simulink model "min_max"  (Simulink 7.4)
settings: Solver=ode45  StartTime=0.0  StopTime=10.0  RelTol=1e-3
libraries: xbsIndex_r4 x38
settings Model: Creator=andryc  LastModifiedBy=andryc

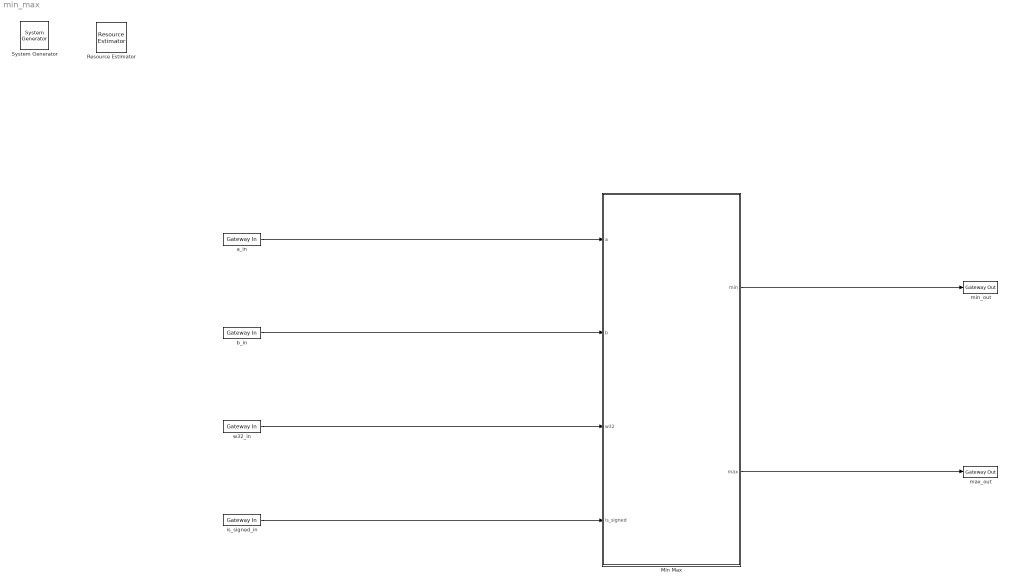
== system min_max ==
  " System Generator" : xbsIndex_r4/ System Generator  Tag=genX  SystemSampleTime=-1  xilinxfamily=virtex5  part=xc5vlx330t  speed=-1  package=ff1738  synthesis_tool=XST  clock_wrapper=Clock Enables  directory=./ngc_netlist  testbench=off  simulink_period=1  sysclk_period=3.333333333  dcm_input_clock_period=10  incr_netlist=off  trim_vbits=Everywhere in SubSystem  dbl_ovrd=According to Block Masks  core_generation=According to Block Masks  run_coregen=off  deprecated_control=off  eval_field=0  block_type=sysgen
  Min Max : Subsystem
  Resource Estimator : xbsIndex_r4/Resource Estimator  Tag=resEstTag  Slices=0  FFs=0  BRAMs=0  LUTs=0  IOBs=0  EBMs=0  TBUFs=0  xl_use_estimator_area=off  est_options=Estimate  block_type=resource_estimator
      settings: AttributesFormatString=Resource\nEstimator
  a_in : xbsIndex_r4/Gateway In  arith_type=Unsigned  n_bits=32  bin_pt=0  quantization=Truncate  overflow=Saturate  period=1  dbl_ovrd=off  timing_constraint=None  locs_specified=off  LOCs={}  hdl_port=on  block_type=gatewayin
      settings: infoedit="Gateway in block.  Converts inputs of type Simulink integer, double and fixed point to  Xilinx fixed point type.<br><br>Hardware notes:  In hardware these blocks become top level input ports."
  b_in : xbsIndex_r4/Gateway In  arith_type=Unsigned  n_bits=32  bin_pt=0  quantization=Truncate  overflow=Saturate  period=1  dbl_ovrd=off  timing_constraint=None  locs_specified=off  LOCs={}  hdl_port=on  block_type=gatewayin
      settings: infoedit="Gateway in block.  Converts inputs of type Simulink integer, double and fixed point to  Xilinx fixed point type.<br><br>Hardware notes:  In hardware these blocks become top level input ports."
  is_signed_in : xbsIndex_r4/Gateway In  arith_type=Unsigned  n_bits=1  bin_pt=0  quantization=Truncate  overflow=Saturate  period=1  dbl_ovrd=off  timing_constraint=None  locs_specified=off  LOCs={}  hdl_port=on  block_type=gatewayin
      settings: infoedit="Gateway in block.  Converts inputs of type Simulink integer, double and fixed point to  Xilinx fixed point type.<br><br>Hardware notes:  In hardware these blocks become top level input ports."
  max_out : xbsIndex_r4/Gateway Out  hdl_port=on  timing_constraint=None  locs_specified=off  LOCs={}  block_type=gatewayout
      settings: infoedit="Gateway out block.  Converts Xilinx fixed point inputs into ouputs of type Simulink integer, double, or fixed point.<br><br>Hardware notes:  In hardware these blocks become top level output ports or are discarded, depending on how they are configured."
  min_out : xbsIndex_r4/Gateway Out  hdl_port=on  timing_constraint=None  locs_specified=off  LOCs={}  block_type=gatewayout
      settings: infoedit="Gateway out block.  Converts Xilinx fixed point inputs into ouputs of type Simulink integer, double, or fixed point.<br><br>Hardware notes:  In hardware these blocks become top level output ports or are discarded, depending on how they are configured."
  w32_in : xbsIndex_r4/Gateway In  arith_type=Unsigned  n_bits=1  bin_pt=0  quantization=Truncate  overflow=Saturate  period=1  dbl_ovrd=off  timing_constraint=None  locs_specified=off  LOCs={}  hdl_port=on  block_type=gatewayin
      settings: infoedit="Gateway in block.  Converts inputs of type Simulink integer, double and fixed point to  Xilinx fixed point type.<br><br>Hardware notes:  In hardware these blocks become top level input ports."
  wires:
  a_in/1 -> Min Max/1(a)
  b_in/1 -> Min Max/2(b)
  w32_in/1 -> Min Max/3(w32)
  is_signed_in/1 -> Min Max/4(is_signed)
  Min Max/2(max) -> max_out/1
  Min Max/1(min) -> min_out/1

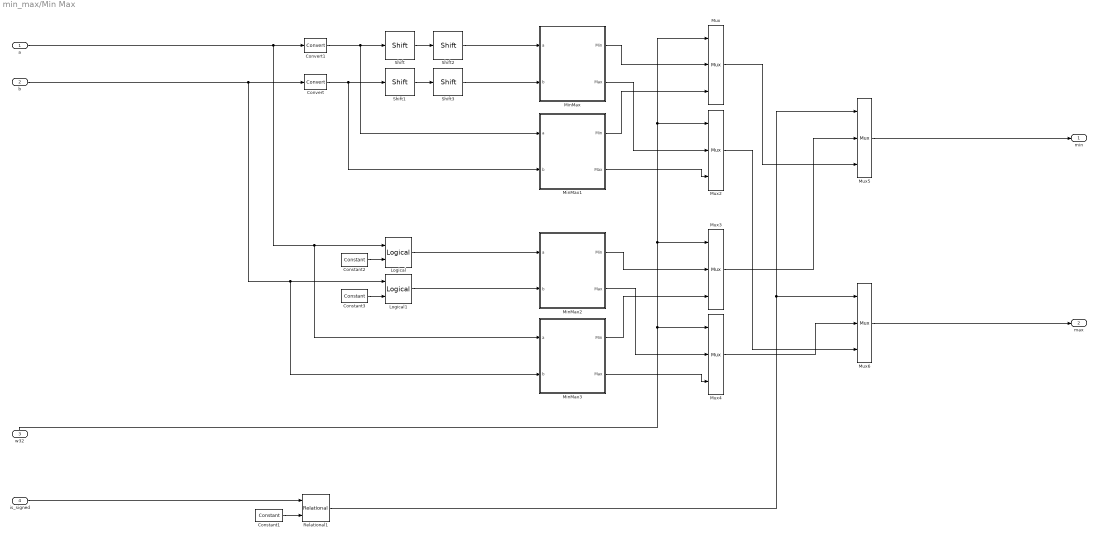
== system min_max/Min Max ==
  a : Inport
  b : Inport  Port=2
  w32 : Inport  Port=3
  is_signed : Inport  Port=4
  Constant1 : xbsIndex_r4/Constant  arith_type=Unsigned  const=1  n_bits=1  bin_pt=0  explicit_period=off  period=1  equ=P=C  opselect=C  inp2=PCIN>>17  opr=+  inp1=P  carry=CIN  dbl_ovrd=off  block_type=constant
      settings: block_version=12.2
  Constant2 : xbsIndex_r4/Constant  arith_type=Unsigned  const=65535  n_bits=32  bin_pt=0  explicit_period=off  period=1  equ=P=C  opselect=C  inp2=PCIN>>17  opr=+  inp1=P  carry=CIN  dbl_ovrd=off  block_type=constant
      settings: block_version=12.2
  Constant3 : xbsIndex_r4/Constant  arith_type=Unsigned  const=65535  n_bits=32  bin_pt=0  explicit_period=off  period=1  equ=P=C  opselect=C  inp2=PCIN>>17  opr=+  inp1=P  carry=CIN  dbl_ovrd=off  block_type=constant
      settings: block_version=12.2
  Convert : xbsIndex_r4/Convert  arith_type="Signed  (2's comp)"  n_bits=31  bin_pt=0  quantization=Truncate  overflow=Saturate  en=off  latency=0  dbl_ovrd=off  pipeline=off  block_type=convert
      settings: block_version=12.2
  Convert1 : xbsIndex_r4/Convert  arith_type="Signed  (2's comp)"  n_bits=32  bin_pt=0  quantization=Truncate  overflow=Saturate  en=off  latency=0  dbl_ovrd=off  pipeline=off  block_type=convert
      settings: block_version=12.2
  Logical : xbsIndex_r4/Logical  logical_function=AND  inputs=2  en=off  latency=0  precision=User Defined  arith_type=Unsigned  n_bits=32  bin_pt=0  align_bp=on  dbl_ovrd=off  block_type=logical
      settings: block_version=12.2
  Logical1 : xbsIndex_r4/Logical  logical_function=AND  inputs=2  en=off  latency=0  precision=User Defined  arith_type=Unsigned  n_bits=32  bin_pt=0  align_bp=on  dbl_ovrd=off  block_type=logical
      settings: block_version=12.2
  MinMax : Subsystem
  MinMax1 : Subsystem
  MinMax2 : Subsystem
  MinMax3 : Subsystem
  Mux{,2..4} (4 alike) : xbsIndex_r4/Mux  inputs=2  en=off  latency=0  precision=Full  arith_type=Unsigned  n_bits=16  bin_pt=14  quantization=Truncate  overflow=Wrap  dbl_ovrd=off  block_type=mux
      settings: block_version=12.2
  Mux5 : xbsIndex_r4/Mux  inputs=2  en=off  latency=0  precision=User Defined  arith_type="Signed  (2's comp)"  n_bits=32  bin_pt=0  quantization=Truncate  overflow=Saturate  dbl_ovrd=off  block_type=mux
      settings: block_version=12.2
  Mux6 : xbsIndex_r4/Mux  inputs=2  en=off  latency=0  precision=User Defined  arith_type=Unsigned  n_bits=32  bin_pt=0  quantization=Truncate  overflow=Saturate  dbl_ovrd=off  block_type=mux
      settings: block_version=12.2
  Relational1 : xbsIndex_r4/Relational  mode=a=b  en=off  latency=0  dbl_ovrd=off  block_type=relational
      settings: block_version=12.2
  Shift : xbsIndex_r4/Shift  shift_dir=Left  shift_bits=16  en=off  latency=0  precision=Full  arith_type="Signed  (2's comp)"  n_bits=31  bin_pt=0  quantization=Truncate  overflow=Saturate  dbl_ovrd=off  block_type=shift
      settings: block_version=12.2
  Shift1 : xbsIndex_r4/Shift  shift_dir=Left  shift_bits=16  en=off  latency=0  precision=Full  arith_type="Signed  (2's comp)"  n_bits=31  bin_pt=0  quantization=Truncate  overflow=Saturate  dbl_ovrd=off  block_type=shift
      settings: block_version=12.2
  Shift2 : xbsIndex_r4/Shift  shift_dir=Right  shift_bits=16  en=off  latency=0  precision=Full  arith_type="Signed  (2's comp)"  n_bits=31  bin_pt=0  quantization=Truncate  overflow=Saturate  dbl_ovrd=off  block_type=shift
      settings: block_version=12.2
  Shift3 : xbsIndex_r4/Shift  shift_dir=Right  shift_bits=16  en=off  latency=0  precision=Full  arith_type="Signed  (2's comp)"  n_bits=31  bin_pt=0  quantization=Truncate  overflow=Saturate  dbl_ovrd=off  block_type=shift
      settings: block_version=12.2
  min : Outport
  max : Outport  Port=2
  wires:
  Constant1/1 -> Relational1/2
  b/1 -> Convert/1, Logical1/1, MinMax3/2(b)
  a/1 -> Convert1/1, Logical/1, MinMax3/1(a)
  Convert1/1 -> Shift/1, MinMax1/1(a)
  Convert/1 -> Shift1/1, MinMax1/2(b)
  Shift1/1 -> Shift3/1
  Shift/1 -> Shift2/1
  Shift2/1 -> MinMax/1(a)
  Shift3/1 -> MinMax/2(b)
  w32/1 -> Mux/1, Mux2/1, Mux3/1, Mux4/1
  MinMax/1(Min) -> Mux/2
  MinMax1/1(Min) -> Mux/3
  MinMax/2(Max) -> Mux2/2
  MinMax1/2(Max) -> Mux2/3
  Constant2/1 -> Logical/2
  Constant3/1 -> Logical1/2
  Logical/1 -> MinMax2/1(a)
  Logical1/1 -> MinMax2/2(b)
  MinMax2/1(Min) -> Mux3/2
  MinMax3/1(Min) -> Mux3/3
  MinMax2/2(Max) -> Mux4/2
  MinMax3/2(Max) -> Mux4/3
  Relational1/1 -> Mux5/1, Mux6/1
  Mux/1 -> Mux5/3
  Mux2/1 -> Mux6/3
  Mux3/1 -> Mux5/2
  Mux4/1 -> Mux6/2
  Mux5/1 -> min/1
  Mux6/1 -> max/1
  is_signed/1 -> Relational1/1

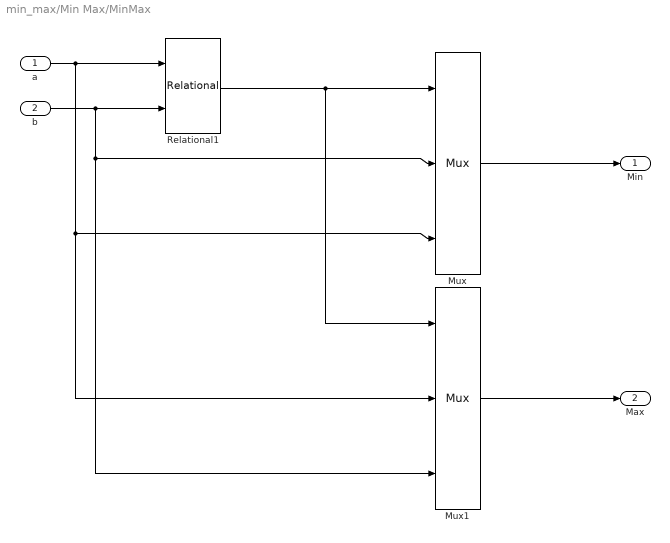
== system min_max/Min Max/MinMax ==
  a : Inport
  b : Inport  Port=2
  Mux : xbsIndex_r4/Mux  inputs=2  en=off  latency=0  precision=Full  arith_type=Unsigned  n_bits=16  bin_pt=14  quantization=Truncate  overflow=Wrap  dbl_ovrd=off  block_type=mux
      settings: block_version=12.2
  Mux1 : xbsIndex_r4/Mux  inputs=2  en=off  latency=0  precision=Full  arith_type=Unsigned  n_bits=16  bin_pt=14  quantization=Truncate  overflow=Wrap  dbl_ovrd=off  block_type=mux
      settings: block_version=12.2
  Relational1 : xbsIndex_r4/Relational  mode=a<=b  en=off  latency=0  dbl_ovrd=off  block_type=relational
      settings: block_version=12.2
  Min : Outport
  Max : Outport  Port=2
  wires:
  Relational1/1 -> Mux/1, Mux1/1
  a/1 -> Relational1/1, Mux/3, Mux1/2
  b/1 -> Relational1/2, Mux/2, Mux1/3
  Mux/1 -> Min/1
  Mux1/1 -> Max/1

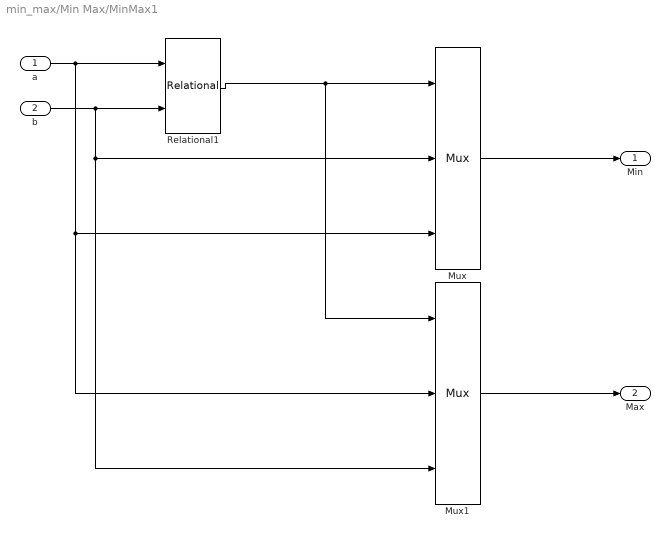
== system min_max/Min Max/MinMax1 ==
  a : Inport
  b : Inport  Port=2
  Mux : xbsIndex_r4/Mux  inputs=2  en=off  latency=0  precision=Full  arith_type=Unsigned  n_bits=16  bin_pt=14  quantization=Truncate  overflow=Wrap  dbl_ovrd=off  block_type=mux
      settings: block_version=12.2
  Mux1 : xbsIndex_r4/Mux  inputs=2  en=off  latency=0  precision=Full  arith_type=Unsigned  n_bits=16  bin_pt=14  quantization=Truncate  overflow=Wrap  dbl_ovrd=off  block_type=mux
      settings: block_version=12.2
  Relational1 : xbsIndex_r4/Relational  mode=a<=b  en=off  latency=0  dbl_ovrd=off  block_type=relational
      settings: block_version=12.2
  Min : Outport
  Max : Outport  Port=2
  wires:
  Mux1/1 -> Max/1
  Mux/1 -> Min/1
  b/1 -> Mux1/3, Mux/2, Relational1/2
  a/1 -> Mux1/2, Mux/3, Relational1/1
  Relational1/1 -> Mux1/1, Mux/1

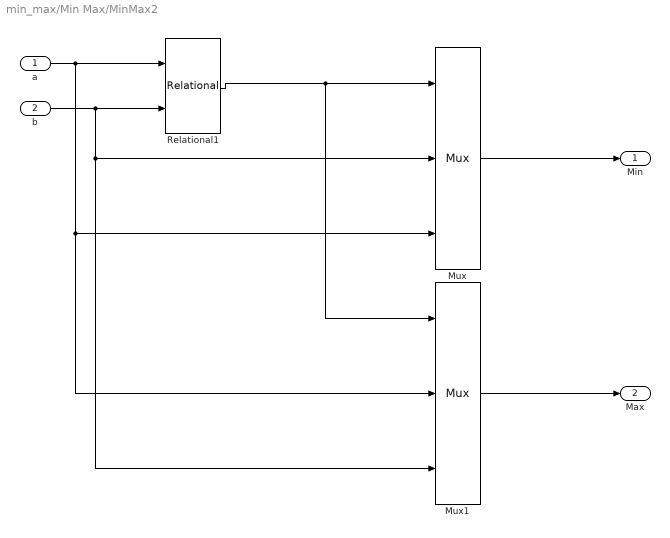
== system min_max/Min Max/MinMax2 ==
  a : Inport
  b : Inport  Port=2
  Mux : xbsIndex_r4/Mux  inputs=2  en=off  latency=0  precision=Full  arith_type=Unsigned  n_bits=16  bin_pt=14  quantization=Truncate  overflow=Wrap  dbl_ovrd=off  block_type=mux
      settings: block_version=12.2
  Mux1 : xbsIndex_r4/Mux  inputs=2  en=off  latency=0  precision=Full  arith_type=Unsigned  n_bits=16  bin_pt=14  quantization=Truncate  overflow=Wrap  dbl_ovrd=off  block_type=mux
      settings: block_version=12.2
  Relational1 : xbsIndex_r4/Relational  mode=a<=b  en=off  latency=0  dbl_ovrd=off  block_type=relational
      settings: block_version=12.2
  Min : Outport
  Max : Outport  Port=2
  wires:
  Relational1/1 -> Mux/1, Mux1/1
  a/1 -> Relational1/1, Mux/3, Mux1/2
  b/1 -> Relational1/2, Mux/2, Mux1/3
  Mux/1 -> Min/1
  Mux1/1 -> Max/1

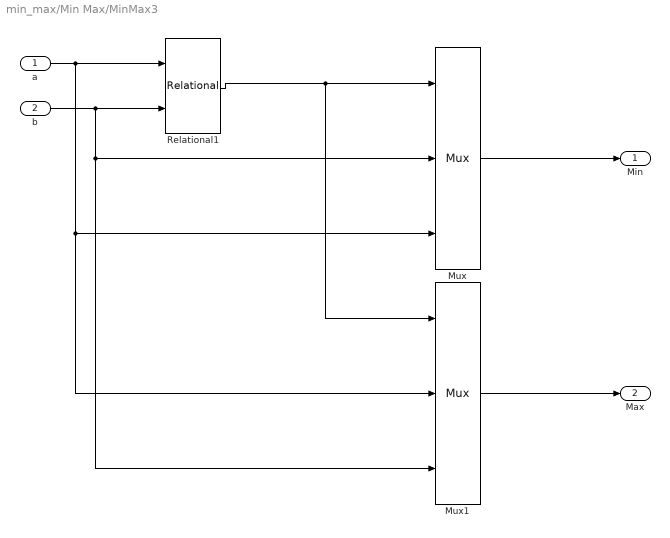
== system min_max/Min Max/MinMax3 ==
  a : Inport
  b : Inport  Port=2
  Mux : xbsIndex_r4/Mux  inputs=2  en=off  latency=0  precision=Full  arith_type=Unsigned  n_bits=16  bin_pt=14  quantization=Truncate  overflow=Wrap  dbl_ovrd=off  block_type=mux
      settings: block_version=12.2
  Mux1 : xbsIndex_r4/Mux  inputs=2  en=off  latency=0  precision=Full  arith_type=Unsigned  n_bits=16  bin_pt=14  quantization=Truncate  overflow=Wrap  dbl_ovrd=off  block_type=mux
      settings: block_version=12.2
  Relational1 : xbsIndex_r4/Relational  mode=a<=b  en=off  latency=0  dbl_ovrd=off  block_type=relational
      settings: block_version=12.2
  Min : Outport
  Max : Outport  Port=2
  wires:
  Mux1/1 -> Max/1
  Mux/1 -> Min/1
  b/1 -> Mux1/3, Mux/2, Relational1/2
  a/1 -> Mux1/2, Mux/3, Relational1/1
  Relational1/1 -> Mux1/1, Mux/1
